simulink model "modele.original"  (R2025b)
settings: Solver=VariableStepAuto  StartTime=0.0  StopTime=20  RelTol=1e-3
values from neighbouring files (symbols this model uses):
  Axy = 0.0    (= 0)    [PropKtKq.m]    (also in variables_procom.m = prop.Axy)
  B = 0    [variables_procom.m]
  Cxy = 0.0    (= 0)    [PropKtKq.m]    (also in variables_procom.m = prop.Cxy)
  D = 0.0    (= 0)    [PropKtKq.m]    (also in variables_procom.m = prop.D)
  Jprop = Jm/Rm^2    (= 18.6702)    [variables_procom.m]
  Ki = 0.1    [variables_procom.m]
  Kim = 60    [variables_procom.m]
  Kp = 3    [variables_procom.m]
  Kpm = 0    [variables_procom.m]
  m = 0.0    (= 0)    [Hulldyn.m]    (also in variables_procom.m = 250000)
  ma = 123434    [variables_procom.m]
  Pe = 5    [variables_procom.m]
  Py = 60    [variables_procom.m]
  Rm = 1/2.9    (= 0.344827586207)    [variables_procom.m]
  tau_f = 0.2    [variables_procom.m]
  Tc = 0.0    (= 0)    [Hulldyn.m]    (also in variables_procom.m = 58000)
  th = 0.0    (= 0)    [Hulldyn.m]    (also in PropKtKq.m; variables_procom.m = hull.th)
  wh = 0.0    (= 0)    [Hulldyn.m]    (also in PropKtKq.m; variables_procom.m = hull.wh)
  x = 0.0    (= 0)    [PropKtKq.m]    (also in variables_procom.m = prop.x)
  y = 0.0    (= 0)    [PropKtKq.m]    (also in variables_procom.m = prop.y)
undefined symbols (not defined in the file or in its folder): kd
libraries: slpidlib x2
settings Model: Creator=leagr  LastModifiedBy=f23berge

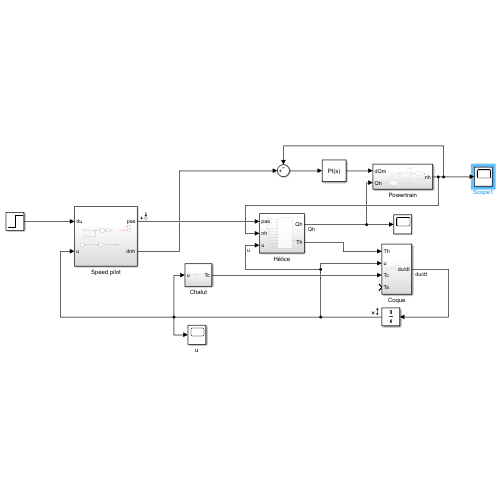
[thumbnail: Simulink's stored preview of the top-level diagram]
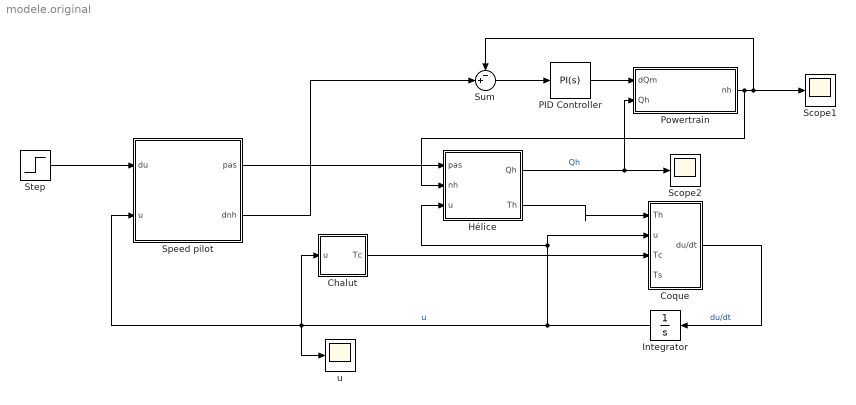
== system modele.original ==
  Chalut : Subsystem
  Coque : Subsystem
  Hélice : Subsystem
  Integrator : Integrator
  PID Controller : slpidlib/PID Controller  Controller=PI  Form=Parallel  TimeDomain=Continuous-time  UseExternalTs=off  SampleTime=-1  IntegratorMethod=Forward Euler  FilterMethod=Forward Euler  ControllerParametersSource=internal  P=Kpm  I=Kim  UseKiTs=off  D=0  UseExternalDerivativeSource=off  N=100  UseFilter=on  TunerSelectOption=Transfer Function Based (PID Tuner App)  InitialConditionSource=internal  InitialConditionForIntegrator=0  InitialConditionForFilter=0  DifferentiatorICPrevScaledInput=0  ExternalReset=none  TrackingMode=off  Kt=1  LimitOutput=off  SatLimitsSource=internal  UpperSaturationLimit=inf  LowerSaturationLimit=-inf  LinearizeAsGain=on  AntiWindupMode=none  Kb=1  LimitIntegrator=off  UpperIntegratorSaturationLimit=inf  LowerIntegratorSaturationLimit=-inf  POutMin=[]  POutMax=[]  IOutMin=[]  IOutMax=[]  DOutMin=[]  DOutMax=[]  NOutMin=[]  NOutMax=[]  SumOutMin=[]  SumOutMax=[]  SaturationOutMin=[]  SaturationOutMax=[]  PParamMin=[]  PParamMax=[]  IParamMin=[]  IParamMax=[]  DParamMin=[]  DParamMax=[]  NParamMin=[]  NParamMax=[]  KbParamMin=[]  KbParamMax=[]  KtParamMin=[]  KtParamMax=[]  KbOutMin=[]  KbOutMax=[]  KtOutMin=[]  KtOutMax=[]  IntegratorOutMin=[]  IntegratorOutMax=[]  FilterOutMin=[]  FilterOutMax=[]  SumI1OutMin=[]  SumI1OutMax=[]  SumI2OutMin=[]  SumI2OutMax=[]  SumI3OutMin=[]  SumI3OutMax=[]  SumI4OutMin=[]  SumI4OutMax=[]  SumDOutMin=[]  SumDOutMax=[]  DifferentiatorOutMin=[]  DifferentiatorOutMax=[]  FilterDiffOutCoefMin=[]  FilterDiffOutCoefMax=[]  ReciprocalOutMin=[]  ReciprocalOutMax=[]  SumDenOutMin=[]  SumDenOutMax=[]  SumNumOutMin=[]  SumNumOutMax=[]  DivideOutMin=[]  DivideOutMax=[]  UdiffTsProdOutMin=[]  UdiffTsProdOutMax=[]  NTsProdOutMin=[]  NTsProdOutMax=[]  UintegralTsProdOutMin=[]  UintegralTsProdOutMax=[]  UngainTsProdOutMin=[]  UngainTsProdOutMax=[]  ClampingZeroOutDataTypeStr=Inherit: Inherit via back propagation  ClampingZeroOutMin=[]  ClampingZeroOutMax=[]  FilterDenConstantOutDataTypeStr=Inherit: Inherit via back propagation  FilterDenConstantOutMin=[]  FilterDenConstantOutMax=[]  PCopyOutDataTypeStr=Inherit: Inherit via back propagation  PCopyOutMin=[]  PCopyOutMax=[]  NCopyOutDataTypeStr=Inherit: Inherit via back propagation  NCopyOutMin=[]  NCopyOutMax=[]  IntegratorContinuousStateAttributes=''  IntegratorStateMustResolveToSignalObject=off  IntegratorRTWStateStorageClass=Auto  FilterContinuousStateAttributes=''  FilterStateMustResolveToSignalObject=off  FilterRTWStateStorageClass=Auto  ParallelPVariant=InternalParameters  IdealPVariant=Disabled  IVariant=InternalParameters  DVariant=Disabled  IntegratorVariant=Continuous  SatVariant=Disabled  AWVariant=Passthrough  PCopyVariant=Disabled  TRVariant=Disabled  FdbkBlocksVariant=Forward  IdealPFdbkVariant=Disabled  SatFdbkVariant=Disabled  DerivativeFilterVariant=Disabled  NVariant=Disabled  NCopyVariant=Disabled_SignalSpec  FilterICVariant=Disabled  IntegratorICVariant=InternalICs  ExternalResetVariant=Disabled  TRSumVariant=Passthrough  SumFdbkVariant=Disabled  SumVariant=Sum_PI  TsampFilterVariant=InternalTs  TsampNgainVariant=Passthrough  TsampIntegralVariant=Disabled_SignalSpec  ExternalSaturationOutDataTypeStr=Inherit: Same as second input  DerivativeSourceVariant=Disabled  PreIntVariant=InternalPreInt
  Powertrain : Subsystem
  Scope1 : Scope
      settings: ActiveDisplayYMinimum=-191.94628532868802  ActiveDisplayYMaximum=391.51178675573277  DataLoggingVariableName=ScopeData3
  Scope2 : Scope
      settings: ActiveDisplayYMinimum=-2.943868322567603E+7  ActiveDisplayYMaximum=8.7335421364796013E+7  DataLoggingVariableName=ScopeData6
  Speed pilot : Subsystem
  Step : Step  Time=10  After=5  SampleTime=0
  Sum : Sum  Inputs=-+|
  u : Scope
      settings: ActiveDisplayYMinimum=-164.07842890826069  ActiveDisplayYMaximum=1476.7058601743465
  wires:
  Sum/1 -> PID Controller/1
  PID Controller/1 -> Powertrain/1(dQm)
  Chalut/1(Tc) -> Coque/3(Tc)
  Powertrain/1(nh) -> Scope1/1, Sum/1, Hélice/2(nh)
  Hélice/1(Qh) -> Powertrain/2(Qh), Scope2/1  "Qh"
  Hélice/2(Th) -> Coque/1(Th)
  Integrator/1 -> Speed pilot/2(u), Chalut/1(u), u/1, Coque/2(u), Hélice/3(u)  "u"
  Coque/1(du/dt) -> Integrator/1  "du/dt"
  Speed pilot/2(dnh) -> Sum/2
  Speed pilot/1(pas) -> Hélice/1(pas)
  Step/1 -> Speed pilot/1(du)

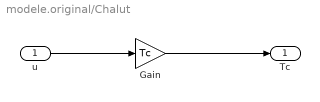
== system modele.original/Chalut ==
  u : Inport
  Gain : Gain  Gain=Tc
  Tc : Outport
  wires:
  u/1 -> Gain/1
  Gain/1 -> Tc/1

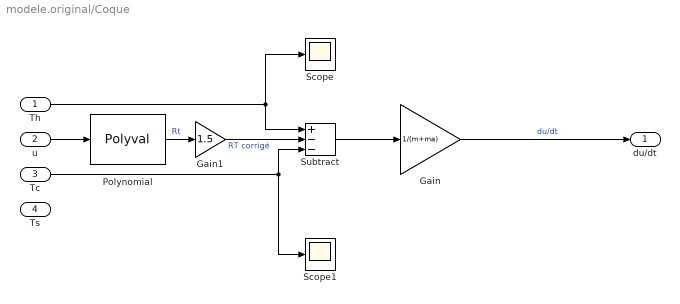
== system modele.original/Coque ==
  Th : Inport
  u : Inport  Port=2
  Tc : Inport  Port=3
  Ts : Inport  Port=4
  Gain : Gain  Gain=1/(m+ma)
  Gain1 : Gain  Gain=1.5
  Polynomial : Polyval  Coefs=[768.9,-3894,6949.8,-271.6]
  Scope : Scope
      settings: ActiveDisplayYMinimum=-1  ActiveDisplayYMaximum=1
  Scope1 : Scope
      settings: ActiveDisplayYMinimum=-1  ActiveDisplayYMaximum=1  DataLoggingVariableName=ScopeData2
  Subtract : Sum  Inputs=+--
  du/dt : Outport
  wires:
  Subtract/1 -> Gain/1
  Polynomial/1 -> Gain1/1  "Rt"
  Tc/1 -> Scope1/1, Subtract/3
  Gain/1 -> du/dt/1  "du/dt"
  Gain1/1 -> Subtract/2  "RT corrigé"
  u/1 -> Polynomial/1
  Th/1 -> Subtract/1, Scope/1

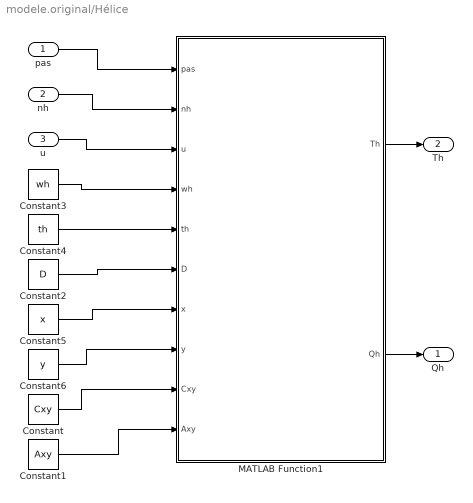
== system modele.original/Hélice ==
  pas : Inport
  nh : Inport  Port=2
  u : Inport  Port=3
  Constant : Constant  Value=Cxy
  Constant1 : Constant  Value=Axy
  Constant2 : Constant  Value=D
  Constant3 : Constant  Value=wh
  Constant4 : Constant  Value=th
  Constant5 : Constant  Value=x
  Constant6 : Constant  Value=y
  MATLAB Function1 : MATLAB Function  TreatAsAtomicUnit=on
  Qh : Outport
  Th : Outport  Port=2
  wires:
  pas/1 -> MATLAB Function1/1(pas)
  nh/1 -> MATLAB Function1/2(nh)
  Constant/1 -> MATLAB Function1/9(Cxy)
  u/1 -> MATLAB Function1/3(u)
  Constant3/1 -> MATLAB Function1/4(wh)
  Constant4/1 -> MATLAB Function1/5(th)
  Constant1/1 -> MATLAB Function1/10(Axy)
  Constant2/1 -> MATLAB Function1/6(D)
  Constant5/1 -> MATLAB Function1/7(x)
  Constant6/1 -> MATLAB Function1/8(y)
  MATLAB Function1/2(Qh) -> Qh/1
  MATLAB Function1/1(Th) -> Th/1

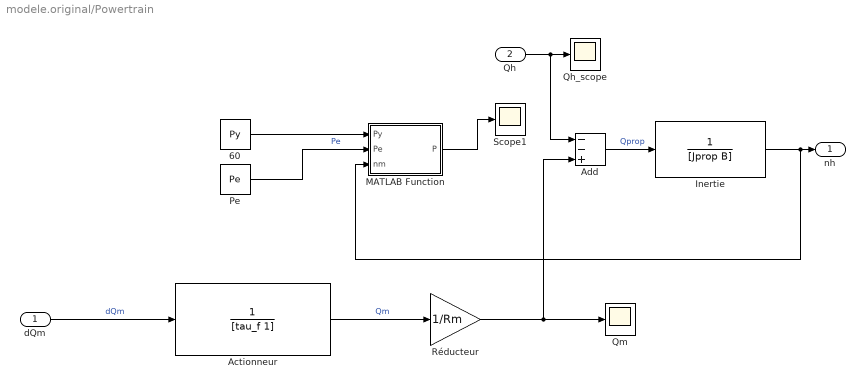
== system modele.original/Powertrain ==
  dQm : Inport
  Qh : Inport  Port=2
  60 : Constant  Value=Py
  Actionneur : TransferFcn  Denominator=[tau_f 1]
  Add : Sum  Inputs=--+
  Inertie : TransferFcn  Denominator=[Jprop B]
  MATLAB Function : MATLAB Function  TreatAsAtomicUnit=on
  Pe : Constant  Value=Pe
  Qh_scope : Scope
      settings: ActiveDisplayYMinimum=-1789.9544650918788  ActiveDisplayYMaximum=14615.425891366995  DataLoggingVariableName=ScopeData4
  Qm : Scope
      settings: ActiveDisplayYMinimum=-1  ActiveDisplayYMaximum=1
  Réducteur : Gain  Gain=1/Rm
  Scope1 : Scope
      settings: ActiveDisplayYMinimum=-1  ActiveDisplayYMaximum=1  DataLoggingVariableName=ScopeData2
  nh : Outport
  wires:
  Qh/1 -> Qh_scope/1, Add/1
  Add/1 -> Inertie/1  "Qprop"
  Réducteur/1 -> Qm/1, Add/3
  Actionneur/1 -> Réducteur/1  "Qm"
  dQm/1 -> Actionneur/1  "dQm"
  Inertie/1 -> MATLAB Function/3(nm), nh/1
  60/1 -> MATLAB Function/1(Py)
  Pe/1 -> MATLAB Function/2(Pe)  "Pe"
  MATLAB Function/1(P) -> Scope1/1

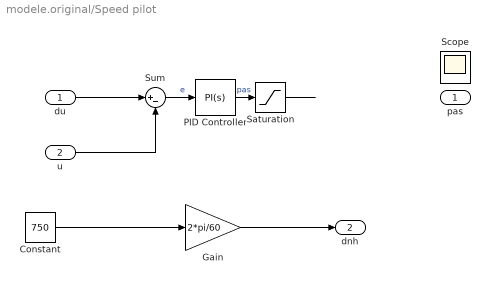
== system modele.original/Speed pilot ==
  du : Inport
  u : Inport  Port=2
  Constant : Constant  Value=750
  Gain : Gain  Gain=2*pi/60
  PID Controller : slpidlib/PID Controller  Controller=PI  Form=Parallel  TimeDomain=Continuous-time  UseExternalTs=off  SampleTime=-1  IntegratorMethod=Forward Euler  FilterMethod=Forward Euler  ControllerParametersSource=internal  P=Kp  I=Ki  UseKiTs=off  D=kd  UseExternalDerivativeSource=off  N=100  UseFilter=on  TunerSelectOption=Transfer Function Based (PID Tuner App)  InitialConditionSource=internal  InitialConditionForIntegrator=0  InitialConditionForFilter=0  DifferentiatorICPrevScaledInput=0  ExternalReset=none  TrackingMode=off  Kt=1  LimitOutput=off  SatLimitsSource=internal  UpperSaturationLimit=inf  LowerSaturationLimit=-inf  LinearizeAsGain=on  AntiWindupMode=none  Kb=1  LimitIntegrator=off  UpperIntegratorSaturationLimit=inf  LowerIntegratorSaturationLimit=-inf  POutMin=[]  POutMax=[]  IOutMin=[]  IOutMax=[]  DOutMin=[]  DOutMax=[]  NOutMin=[]  NOutMax=[]  SumOutMin=[]  SumOutMax=[]  SaturationOutMin=[]  SaturationOutMax=[]  PParamMin=[]  PParamMax=[]  IParamMin=[]  IParamMax=[]  DParamMin=[]  DParamMax=[]  NParamMin=[]  NParamMax=[]  KbParamMin=[]  KbParamMax=[]  KtParamMin=[]  KtParamMax=[]  KbOutMin=[]  KbOutMax=[]  KtOutMin=[]  KtOutMax=[]  IntegratorOutMin=[]  IntegratorOutMax=[]  FilterOutMin=[]  FilterOutMax=[]  SumI1OutMin=[]  SumI1OutMax=[]  SumI2OutMin=[]  SumI2OutMax=[]  SumI3OutMin=[]  SumI3OutMax=[]  SumI4OutMin=[]  SumI4OutMax=[]  SumDOutMin=[]  SumDOutMax=[]  DifferentiatorOutMin=[]  DifferentiatorOutMax=[]  FilterDiffOutCoefMin=[]  FilterDiffOutCoefMax=[]  ReciprocalOutMin=[]  ReciprocalOutMax=[]  SumDenOutMin=[]  SumDenOutMax=[]  SumNumOutMin=[]  SumNumOutMax=[]  DivideOutMin=[]  DivideOutMax=[]  UdiffTsProdOutMin=[]  UdiffTsProdOutMax=[]  NTsProdOutMin=[]  NTsProdOutMax=[]  UintegralTsProdOutMin=[]  UintegralTsProdOutMax=[]  UngainTsProdOutMin=[]  UngainTsProdOutMax=[]  ClampingZeroOutDataTypeStr=Inherit: Inherit via back propagation  ClampingZeroOutMin=[]  ClampingZeroOutMax=[]  FilterDenConstantOutDataTypeStr=Inherit: Inherit via back propagation  FilterDenConstantOutMin=[]  FilterDenConstantOutMax=[]  PCopyOutDataTypeStr=Inherit: Inherit via back propagation  PCopyOutMin=[]  PCopyOutMax=[]  NCopyOutDataTypeStr=Inherit: Inherit via back propagation  NCopyOutMin=[]  NCopyOutMax=[]  IntegratorContinuousStateAttributes=''  IntegratorStateMustResolveToSignalObject=off  IntegratorRTWStateStorageClass=Auto  FilterContinuousStateAttributes=''  FilterStateMustResolveToSignalObject=off  FilterRTWStateStorageClass=Auto  ParallelPVariant=InternalParameters  IdealPVariant=Disabled  IVariant=InternalParameters  DVariant=Disabled  IntegratorVariant=Continuous  SatVariant=Disabled  AWVariant=Passthrough  PCopyVariant=Disabled  TRVariant=Disabled  FdbkBlocksVariant=Forward  IdealPFdbkVariant=Disabled  SatFdbkVariant=Disabled  DerivativeFilterVariant=Disabled  NVariant=Disabled  NCopyVariant=Disabled_SignalSpec  FilterICVariant=Disabled  IntegratorICVariant=InternalICs  ExternalResetVariant=Disabled  TRSumVariant=Passthrough  SumFdbkVariant=Disabled  SumVariant=Sum_PI  TsampFilterVariant=InternalTs  TsampNgainVariant=Passthrough  TsampIntegralVariant=Disabled_SignalSpec  ExternalSaturationOutDataTypeStr=Inherit: Same as second input  DerivativeSourceVariant=Disabled  PreIntVariant=InternalPreInt
  Saturation : Saturate  UpperLimit=2  LowerLimit=0
  Scope : Scope
      settings: ActiveDisplayYMinimum=-0.24999999999999994  ActiveDisplayYMaximum=2.25  DataLoggingVariableName=ScopeData5
  Sum : Sum  Inputs=|+-
  pas : Outport
  dnh : Outport  Port=2
  wires:
  u/1 -> Sum/2
  Sum/1 -> PID Controller/1  "e"
  PID Controller/1 -> Saturation/1  "pas"
  du/1 -> Sum/1
  Constant/1 -> Gain/1
  Saturation/1 -> ?
  Gain/1 -> dnh/1
  ? -> Scope/1, pas/1

== matlab function modele.original/Hélice/MATLAB Function1 ==
  data: pas input; nh input; u input; Th output; Qh output; wh input; th input; D input; x input; y input; Cxy input; Axy input
function [Th,Qh]= fcn(pas, nh, u, wh, th ,D, x, y, Cxy, Axy)
    
    % Conversion nh de rad/s vers tr/s
    nh = nh/(2*pi);

    rho = 1025; % Masse volumique de l'eau

    % Coefficient d'avance et rapport P/D
    if pas < 1e-6
        J = 0.8;
    else
        J = u*(1-wh)/(D*nh);
    end
    P_D = pas/D;
        
    % Calcul des coefficients Kt et Kq pour ce point de fonctionnement
    % La cartographie est valide pour P/D dans [0.3; 1.5]
    % et J dans [0; 0.8]      
    J = min(max(J, 0), 0.8);
    P_D = min(max(P_D, 0.3), 1.5);

    Kt = dot(Axy, P_D.^x .* J.^y);
    Kq = dot(Cxy, P_D.^x .* J.^y);
        
    % Calcul de la poussée
    if Kt<0
        Kt=0;
    end
    if Kq<0 || Kq ==0
        Kq = 0.2;
    end
    Th = (1-th)*Kt*rho*D^4*nh^2;
    Qh = Kq*rho*D^5*nh^2;
    
    %if du <= 0
    %    Th = 0;
    %    Qh = 0;
    %end
end

== matlab function modele.original/Powertrain/MATLAB Function ==
  data: Py input; P output; Pe input; nm input
function P = fcn(Py, Pe, nm)
threshold = 40; % On ne branche l'aternateur et les pompes qu'une fois
                 % un certain régime atteint.
eta_p = 0.5;
    if nm < threshold
        P = 0;
    else
        P = (Pe*eta_p+Py)/nm;
    end
